simulink model "ARM_closedloop_real_Serial"  (R2021a)
settings: Solver=VariableStepAuto  StartTime=0.0  StopTime=1500  RelTol=1e-3  EnableMultiTasking=on
StopFcn:
  | clear ARM_lab_realtime_udp;
undefined symbols (not defined in the file): DiscIntNeverNeededParam
libraries: simulink x1, realtime_pacer_lib x1
CloseFcn:
  | clear ARM_lab_realtime_udp;
settings Model: OrderedModelArguments=off  Creator=johnh  LastModifiedBy=Andy
settings SolverCC: AlgebraicLoopSolver=TrustRegion
settings DataIOCC: ReturnWorkspaceOutputs=off
settings OptimizationCC: LifeSpan=inf
settings DebuggingCC: SFUnexpectedBacktrackingDiag=warning  SFNoUnconditionalDefaultTransitionDiag=warning  SFExecutionAtInitializationDiag=none  SFMachineParentedDataDiag=warning  ArithmeticOperatorsInVariantConditions=warning
settings SFSimCC: SimUseLocalCustomCode=off  CustomCodeUndefinedFunction=UseInterfaceOnly
settings RTWCC: RTWUseLocalCustomCode=off
settings CodeAppCC: StateflowObjectComments=on
settings GRTTargetCC: TargetLangStandard=C89/C90 (ANSI)
settings ConfigComp: CovMetricSettings=dw  CovSaveCumulativeToWorkspaceVar=on  CovSaveSingleToWorkspaceVar=on  CovExternalEMLEnable=off

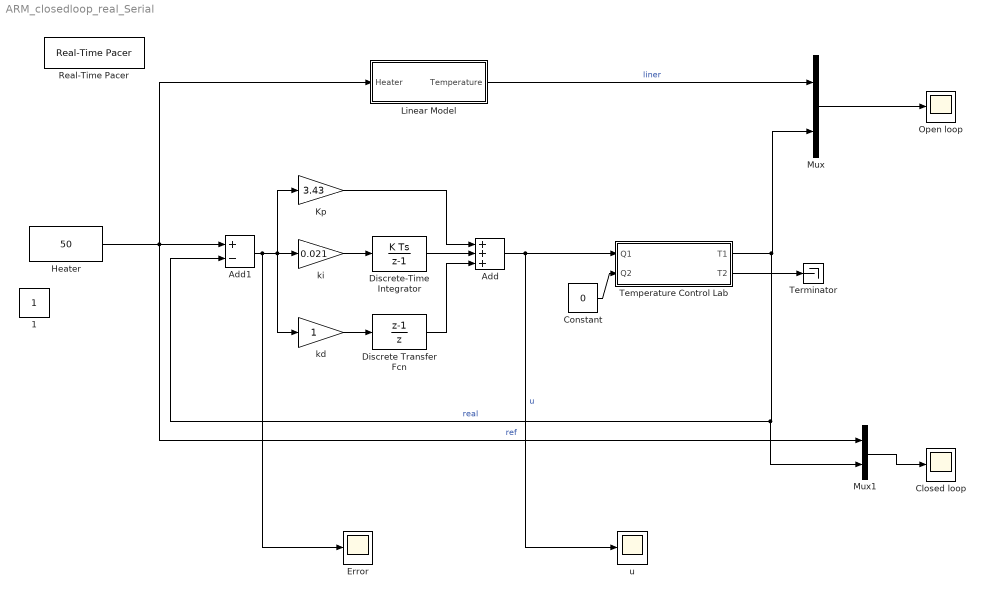
== system ARM_closedloop_real_Serial ==
  Add : Sum  Inputs=+++
  Add1 : Sum  Inputs=+-
  Closed loop : Scope
  Constant : Constant  Value=0
  Discrete Transfer Fcn : DiscreteTransferFcn  Numerator=[1 -1]  Denominator=[1 0]  SampleTime=1
  Discrete-Time Integrator : DiscreteIntegrator  ICPrevOutput=DiscIntNeverNeededParam  ICPrevScaledInput=DiscIntNeverNeededParam
  Error : Scope
  Heater : simulink/Math Operations/Slider Gain  gain=50  low=0  high=120
  Kp : Gain  Gain=3.43
  Linear Model : Subsystem
  Mux : Mux  Inputs=2
  Mux1 : Mux  Inputs=2
  Open loop : Scope
  Real-Time Pacer : realtime_pacer_lib/Real-Time Pacer  simTimePerRealTime=1
  Temperature Control Lab : Subsystem
  Terminator : Terminator
  kd : Gain
  ki : Gain  Gain=0.021
  u : Scope
  1 : Constant  IOType=siggen
  wires:
  Mux/1 -> Open loop/1
  Linear Model/1(Temperature) -> Mux/1  "liner"
  Constant/1 -> Temperature Control Lab/2(Q2)
  Temperature Control Lab/2(T2) -> Terminator/1
  Temperature Control Lab/1(T1) -> Mux1/2, Add1/2, Mux/2  "real"
  ki/1 -> Discrete-Time Integrator/1
  kd/1 -> Discrete Transfer Fcn/1
  Discrete Transfer Fcn/1 -> Add/3
  Discrete-Time Integrator/1 -> Add/2
  Kp/1 -> Add/1
  Add1/1 -> Error/1, Kp/1, kd/1, ki/1
  Add/1 -> u/1, Temperature Control Lab/1(Q1)  "u"
  Mux1/1 -> Closed loop/1
  Heater/1 -> Mux1/1, Add1/1, Linear Model/1(Heater)  "ref"

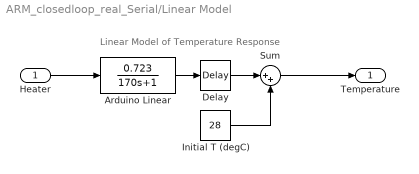
== system ARM_closedloop_real_Serial/Linear Model ==
  note: Linear Model of Temperature Response
  Heater : Inport
  Arduino Linear : TransferFcn  Numerator=[0.723]  Denominator=[170 1]
  Delay : TransportDelay  DelayTime=3
  Initial T (degC) : Constant  Value=28
  Sum : Sum  Inputs=|++
  Temperature : Outport  VectorParamsAs1DForOutWhenUnconnected=off
  wires:
  Arduino Linear/1 -> Delay/1
  Delay/1 -> Sum/1
  Initial T (degC)/1 -> Sum/2
  Sum/1 -> Temperature/1
  Heater/1 -> Arduino Linear/1

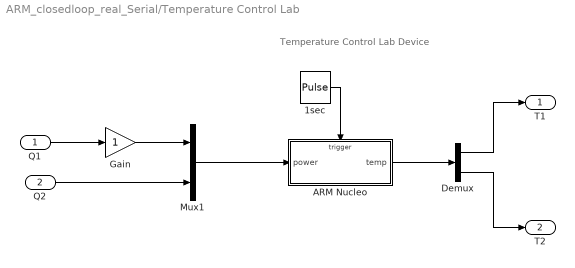
== system ARM_closedloop_real_Serial/Temperature Control Lab ==
  note: Temperature Control Lab Device
  Q1 : Inport
  Q2 : Inport  Port=2
  1sec : DiscretePulseGenerator  PulseType=Time based  Period=1  PulseWidth=50
  ARM Nucleo : Subsystem  TreatAsAtomicUnit=on
  Demux : Demux  Outputs=2
  Gain : Gain
  Mux1 : Mux  Inputs=2
  T1 : Outport  VectorParamsAs1DForOutWhenUnconnected=off
  T2 : Outport  Port=2  VectorParamsAs1DForOutWhenUnconnected=off
  wires:
  1sec/1 -> ARM Nucleo/Trigger
  Mux1/1 -> ARM Nucleo/1(power)
  Q1/1 -> Gain/1
  Q2/1 -> Mux1/2
  Gain/1 -> Mux1/1
  ARM Nucleo/1(temp) -> Demux/1
  Demux/1 -> T1/1
  Demux/2 -> T2/1

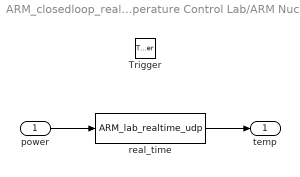
== system ARM_closedloop_real_Serial/Temperature Control Lab/ARM Nucleo ==
  power : Inport  LatchByDelayingOutsideSignal=on
  Trigger : TriggerPort  VariantControl=Variant
  real_time : MATLABFcn  MATLABFcn=ARM_lab_realtime_udp  Output1D=off
  temp : Outport  InitialOutput=25  VectorParamsAs1DForOutWhenUnconnected=off
  wires:
  power/1 -> real_time/1
  real_time/1 -> temp/1
